simulink library "Subchart_FluxMapID_references"  (R2021b)
settings: Solver=VariableStepAuto  StartTime=0.0  StopTime=10.0  RelTol=1e-3
settings Model: Creator=valen  LastModifiedBy=valen

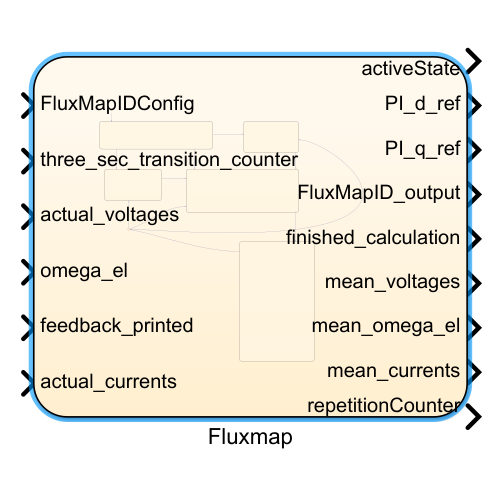
[thumbnail: Simulink's stored preview of the top-level diagram]
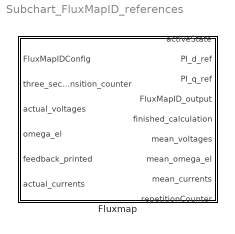
== system Subchart_FluxMapID_references ==
  Fluxmap : Stateflow chart  TreatAsAtomicUnit=on

== stateflow chart Subchart_FluxMapID_references/Fluxmap ==
  settings: executeAtInitialization=1  initializeOutput=1  description=Dampingfactor
  state initAMM
    entry:
    activeState = uint16(401);
    stepsize_d = FluxMapIDConfig.IDstepsize;
    stepsize_q = FluxMapIDConfig.IQstepsize;
    NumberOfIDpoints = uint32(abs(FluxMapIDConfig.IDstop-FluxMapIDConfig.IDstart)/stepsize_d+1);
    NumberOfIQpoints = uint32(abs(FluxMapIDConfig.IQstop-FluxMapIDConfig.IQstart)/stepsize_q+1);
    NumberOfPoints = uint32(NumberOfIDpoints*NumberOfIQpoints);
  state AMMheating
    entry:
    activeState = uint16(420);
  state AMMcooling
    entry:
    activeState = uint16(410);
  state AMMnewRef
    entry:
    counter_time = uint32(1);
    activeState = uint16(402);
    if((FluxMapIDConfig.IDstart + single(AMMn) * stepsize_d) <= FluxMapIDConfig.IDstop)
    PI_d_ref = single(FluxMapIDConfig.IDstart + single(AMMn) * stepsize_d);
    if(mod(single(AMMn),((abs(FluxMapIDConfig.IDstop-FluxMapIDConfig.IDstart))/stepsize_d)+1) == 0)
    if((FluxMapIDConfig.IQstart + single(AMMj) * stepsize_q) <= FluxMapIDConfig.IQstop)
    PI_q_ref = single(FluxMapIDConfig.IQstart + single(AMMj) * stepsize_q);
    AMMj = AMMj + 1;
    else
    PI_d_ref = single(0.75);
    PI_q_ref = single(0.0);
    end
    end
    end
    during: counter_time = counter_time +1;
  state AMMcollectData
    entry:
    counter_time = uint32(1);
    activeState = uint16(403);
    repetitionCounter = repetitionCounter + 1;
    if(AMMn >= (NumberOfIDpoints-1))
    AMMn = uint32(0);
    else
    AMMn = AMMn + 1;
    end
    FluxMapID_output.external_Measurement_Flag=boolean(1);
    during:
    if(i>=array_size+1)
    switch i
    case array_size+1
    mean_voltages.d = mean(u_d_array);
    i = i+1;
    case array_size+2
    mean_voltages.q = mean(u_q_array);
    i = i+1;
    case array_size+3
    mean_omega_el = mean(omega_el_array);
    i = i+1;
    case array_size+4
    mean_currents.d = mean(i_d_array);
    i = i+1;
    case array_size+5
    mean_currents.q = mean(i_q_array);
    i = i+1;
    case array_size+6
    finished_calculation = true;
    i = i+1;
    end
    else
    counter_time = counter_time +1;
    if((mod(counter_time,20)==0)&&i<=array_size)
    i_d_array(i) = actual_currents.d;
    i_q_array(i) = actual_currents.q;
    u_d_array(i) = actual_voltages.d;
    u_q_array(i) = actual_voltages.q;
    omega_el_array(i) = omega_el;
    i = i+1;
    end
    end
    exit:
    FluxMapID_output.external_Measurement_Flag=boolean(0);
    finished_calculation = false;
  (default) -> initAMM
  initAMM -> AMMheating [order 2] : [FluxMapID_output.WindingTemp < FluxMapIDConfig.lower_meas_temp && ....
      | FluxMapIDConfig.start_FM_ID==1]
  (junction 152) -> AMMheating [order 3] : [FluxMapID_output.WindingTemp < FluxMapIDConfig.lower_meas_temp]
  initAMM -> AMMcooling [order 1] : [FluxMapID_output.WindingTemp > FluxMapIDConfig.upper_meas_temp && ....
      | FluxMapIDConfig.start_FM_ID==1]
  initAMM -> AMMnewRef [order 3] : [FluxMapID_output.WindingTemp >=FluxMapIDConfig.lower_meas_temp && ....
      | FluxMapID_output.WindingTemp <=FluxMapIDConfig.upper_meas_temp && ....
      | FluxMapIDConfig.start_FM_ID==1]
  AMMheating -> AMMnewRef : [FluxMapID_output.WindingTemp >= FluxMapIDConfig.lower_meas_temp]
  AMMcooling -> AMMnewRef : [FluxMapID_output.WindingTemp <= FluxMapIDConfig.upper_meas_temp]
  (junction 152) -> AMMcooling [order 1] : [FluxMapID_output.WindingTemp > FluxMapIDConfig.upper_meas_temp]
  (junction 152) -> AMMnewRef [order 2] : [FluxMapID_output.WindingTemp >=FluxMapIDConfig.lower_meas_temp && FluxMapID_output.WindingTemp <= FluxMapIDConfig.upper_meas_temp]
  AMMnewRef -> AMMcollectData : [three_sec_transition_counter == counter_time]
  AMMcollectData -> (junction 152) [order 1] : [(repetitionCounter < NumberOfPoints) && (feedback_printed==true)]
  AMMcollectData -> 164 [order 2] : [(repetitionCounter>=NumberOfPoints) && (feedback_printed==true)]
  data: i_d_ref_AMM_loc local single size=1 =single(0); i_q_ref_AMM_loc local single size=1 =single(0); i_d_ref_AMM_loc local single size=1 =single(0); i_q_ref_AMM_loc local single size=1 =single(0); i local uint32 size=1 =uint32(1); u_d_array local single size=array_size =single(0); u_q_array local single size=array_size =single(0); omega_el_array local single size=array_size =single(0); array_size constant uint16 size=1 =1000; i_d_array local single size=array_size =single(0); i_q_array local single size=array_size =single(0); activeState output uint16 size=1 =uint16(0); PI_d_ref output single size=1; PI_q_ref output single size=1; FluxMapIDConfig input Bus: uz_ParaID_FluxMapIDConfig_t size=1; NumberOfIDpoints local uint32 size=1; NumberOfIQpoints local uint32 size=1; NumberOfPoints local uint32 size=1; counter_time local uint32 size=1; AMMn local uint32 size=1 =uint32(0); AMMj local uint32 size=1 =uint32(0); three_sec_transition_counter input uint32 size=1; FluxMapID_output output Bus: uz_ParaID_FluxMapID_output_t size=1; actual_voltages input Bus: uz_3ph_dq_t size=1; omega_el input single size=1; feedback_printed input boolean size=1; finished_calculation output boolean size=1; mean_voltages output Bus: uz_3ph_dq_t size=1; mean_omega_el output single size=1 =single(0); mean_currents output Bus: uz_3ph_dq_t size=1; repetitionCounter output uint32 size=1 =uint32(0); actual_currents input Bus: uz_3ph_dq_t size=1; stepsize_d local single size=1; stepsize_q local single size=1
  data i_d_ref_AMM_loc settings: description=holds actual setpoints during heating and cooling where specific other setpoints are applied
  data i_q_ref_AMM_loc settings: description=holds actual setpoints during heating and cooling where specific other setpoints are applied
  data i_d_ref_AMM_loc settings: description=holds actual setpoints during heating and cooling where specific other setpoints are applied
  data i_q_ref_AMM_loc settings: description=holds actual setpoints during heating and cooling where specific other setpoints are applied
